simulink model "base_model_1_new - Copy"  (R2025b)
settings: Solver=VariableStepAuto  StartTime=0.0  StopTime=3600  RelTol=1e-3
libraries: fl_lib x4, simulink x2, nesl_utility x1
settings Model: Creator=Gmusl  LastModifiedBy=Collins Addo

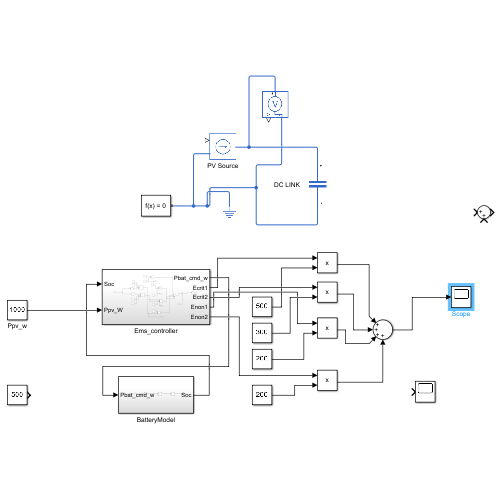
[thumbnail: Simulink's stored preview of the top-level diagram]
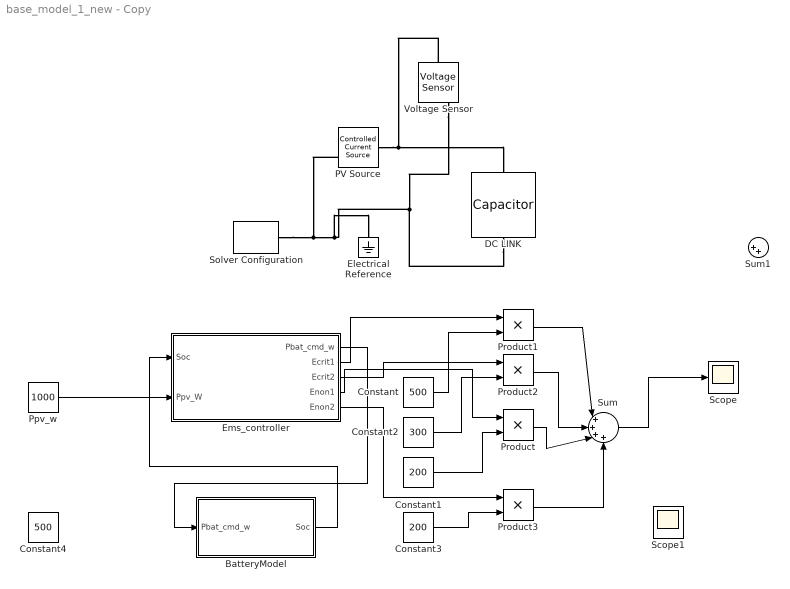
== system base_model_1_new - Copy ==
  BatteryModel : Subsystem
  Constant : Constant  Value=500
  Constant1 : Constant  Value=200
  Constant2 : Constant  Value=300
  Constant3 : Constant  Value=200
  Constant4 : Constant  Value=500
  DC LINK : fl_lib/Electrical/Electrical Elements/Capacitor  c=1e-6 F  r=1e-6 Ohm  g=0 1/Ohm  i_specify=off  i_priority=None  i=0 A  i_nominal_specify=off  i_nominal_value=1  i_nominal_unit=A  v_specify=off  v_priority=None  v=0 V  v_nominal_specify=off  v_nominal_value=1  v_nominal_unit=V  vc_specify=off  vc_priority=High  vc=0 V  vc_nominal_specify=off  vc_nominal_value=1  vc_nominal_unit=V
  Electrical Reference : fl_lib/Electrical/Electrical Elements/Electrical Reference
  Ems_controller : Subsystem
  PV Source : fl_lib/Electrical/Electrical Sources/Controlled Current Source
  Ppv_w : Constant  Value=1000
  Product{,1..3} (4 alike) : Product
  Scope : Scope
      settings: ActiveDisplayYMinimum=0  ActiveDisplayYMaximum=1
  Scope1 : Scope
      settings: ActiveDisplayYMinimum=-0.47972213353852167  ActiveDisplayYMaximum=1.7031524548434163
  Solver Configuration : nesl_utility/Solver Configuration  PhysicalDomain=network_engine_domain  SubClassName=solver  LeftPortType=input  RightPortType=generic  Tones=[]  Harmonics=[]  SimulateNoise=off  Profile=off  UseLocalSampling=off  EnableSwitchedLinearOptims=on  FrequencyDomain=off  UseCCode=off  RelTol=0.001  AbsTol=0.001  MinStep=1e-09  ToWorkspace=off  RevertToSquareIcSolve=off  NumHomotopyIterations=100  PhasorMode=off  PhasorModeNumHarmonics=1  ConsistencySolver=NEWTON_XTOL_AFTER_FTOL  IndexReductionMethod=DerivativeReplacement  DoDC=off  ResidualTolerance=1e-09  ConsistencyTolSource=GLOBAL  ConsistencyAbsTol=0.001  ConsistencyRelTol=0.001  ConsistencyTolFactor=0.001  UseLocalSolver=off  LocalSolverChoice=NE_BACKWARD_EULER_ADVANCER  ResolveIndetEquations=on  FunctionEvalNumThread=1  LocalSolverSampleTime=0.001  DoFixedCost=off  MaxNonlinIter=3  MaxModeIter=2  ComputeImpulses=off  ImpulseIterations=2  LinearAlgebra=auto  LinearAlgebraNumThread=0  EquationFormulation=NE_TIME_EF  DelaysMemoryBudget=1024  AutomaticFiltering=on  FilteringTimeConstant=0.001  PartitionStorageMethod=AS_NEEDED  PartitionMemoryBudget=1024  PartitionMethod=ROBUST  MultibodyUseLocalSolver=off  MultibodyLocalSolverChoice=ODE1  MultibodyLocalSolverSampleTime=0.001
  Sum : Sum  Inputs=|++++
  Sum1 : Sum  Inputs=|++
  Voltage Sensor : fl_lib/Electrical/Electrical Sensors/Voltage Sensor
  wires:
  Ppv_w/1 -> Ems_controller/2(Ppv_W)
  Ems_controller/2(Ecrit1) -> Product1/1
  Constant/1 -> Product1/2
  Ems_controller/3(Ecrit2) -> Product2/1
  Constant2/1 -> Product2/2
  Ems_controller/4(Enon1) -> Product/1
  Constant1/1 -> Product/2
  Ems_controller/5(Enon2) -> Product3/1
  Constant3/1 -> Product3/2
  Product1/1 -> Sum/1
  Product2/1 -> Sum/2
  Product/1 -> Sum/3
  Product3/1 -> Sum/4
  Sum/1 -> Scope/1
  BatteryModel/1(Soc) -> Ems_controller/1(Soc)
  Ems_controller/1(Pbat_cmd_w) -> BatteryModel/1(Pbat_cmd_w)
  connections:
  Solver Configuration/RConn1 -- PV Source/RConn2 -- DC LINK/RConn1 -- Voltage Sensor/RConn2 -- Electrical Reference/LConn1
  PV Source/LConn1 -- Voltage Sensor/LConn1 -- DC LINK/LConn1

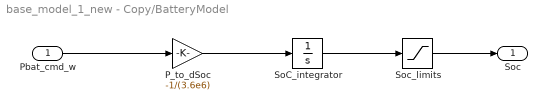
== system base_model_1_new - Copy/BatteryModel ==
  Pbat_cmd_w : Inport
  P_to_dSoc : Gain  Gain=-1/(3.6e6)
  SoC_integrator : Integrator  InitialCondition=0.8
  Soc_limits : Saturate  UpperLimit=0.95  LowerLimit=0.2
  Soc : Outport
  wires:
  Pbat_cmd_w/1 -> P_to_dSoc/1
  P_to_dSoc/1 -> SoC_integrator/1
  SoC_integrator/1 -> Soc_limits/1
  Soc_limits/1 -> Soc/1

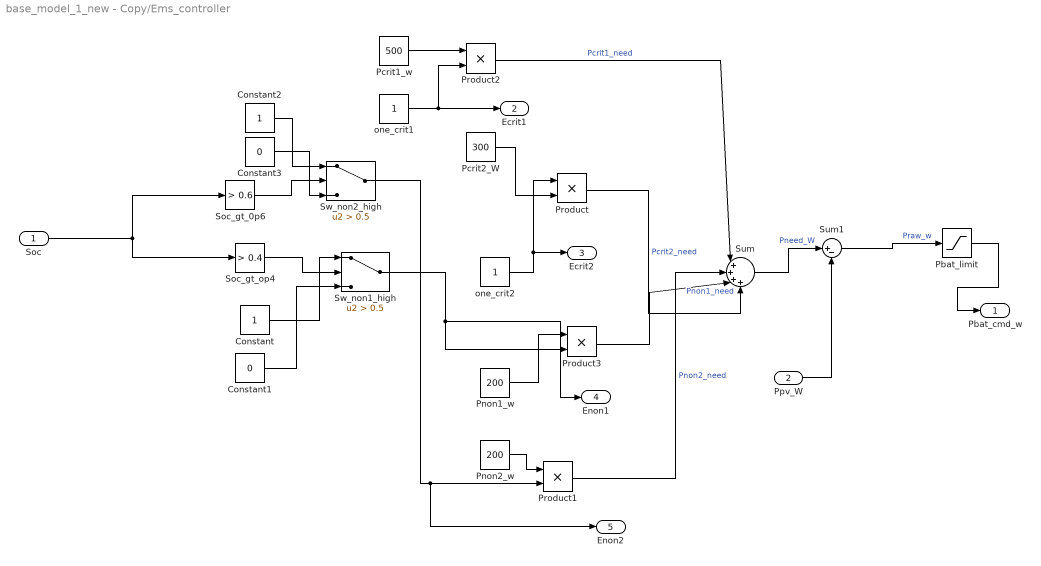
== system base_model_1_new - Copy/Ems_controller ==
  Soc : Inport
  Ppv_W : Inport  Port=2
  Constant : Constant
  Constant1 : Constant  Value=0
  Constant2 : Constant
  Constant3 : Constant  Value=0
  Pbat_limit : Saturate  UpperLimit=2000  LowerLimit=-2000
  Pcrit1_w : Constant  Value=500
  Pcrit2_W : Constant  Value=300
  Pnon1_w : Constant  Value=200
  Pnon2_w : Constant  Value=200
  Product{,1..3} (4 alike) : Product
  Soc_gt_0p6 : simulink/Logic and Bit Operations/Compare To Constant  relop=>  const=0.6  OutDataTypeStr=boolean
  Soc_gt_op4 : simulink/Logic and Bit Operations/Compare To Constant  relop=>  const=0.4  OutDataTypeStr=boolean
  Sum : Sum  Inputs=|++++
  Sum1 : Sum  Inputs=|+-
  Sw_non1_high : Switch  Criteria=u2 > Threshold  Threshold=0.5  SaturateOnIntegerOverflow=off  InputSameDT=off
  Sw_non2_high : Switch  Criteria=u2 > Threshold  Threshold=0.5  SaturateOnIntegerOverflow=off  InputSameDT=off
  one_crit1 : Constant
  one_crit2 : Constant
  Pbat_cmd_w : Outport
  Ecrit1 : Outport  Port=2
  Ecrit2 : Outport  Port=3
  Enon1 : Outport  Port=4
  Enon2 : Outport  Port=5
  wires:
  one_crit1/1 -> Product2/2, Ecrit1/1
  Soc/1 -> Soc_gt_0p6/1, Soc_gt_op4/1
  Soc_gt_op4/1 -> Sw_non1_high/2
  Constant/1 -> Sw_non1_high/1
  Constant1/1 -> Sw_non1_high/3
  Soc_gt_0p6/1 -> Sw_non2_high/2
  Constant3/1 -> Sw_non2_high/3
  Constant2/1 -> Sw_non2_high/1
  Pcrit1_w/1 -> Product2/1
  Product2/1 -> Sum/1  "Pcrit1_need"
  one_crit2/1 -> Product/1, Ecrit2/1
  Pcrit2_W/1 -> Product/2
  Product/1 -> Sum/4  "Pcrit2_need"
  Sw_non1_high/1 -> Enon1/1, Product3/2
  Pnon1_w/1 -> Product3/1
  Product3/1 -> Sum/3  "Pnon1_need"
  Sw_non2_high/1 -> Enon2/1, Product1/2
  Pnon2_w/1 -> Product1/1
  Product1/1 -> Sum/2  "Pnon2_need"
  Sum/1 -> Sum1/1  "Pneed_W"
  Ppv_W/1 -> Sum1/2
  Sum1/1 -> Pbat_limit/1  "Praw_w"
  Pbat_limit/1 -> Pbat_cmd_w/1
